simulink model "Problem3"  (R2020b)
settings: Solver=VariableStepAuto  StartTime=0.0  StopTime=120.0  RelTol=1e-3
settings Model: DataDictionary=Problem3.sldd  Creator=Shirish  LastModifiedBy=Shirish

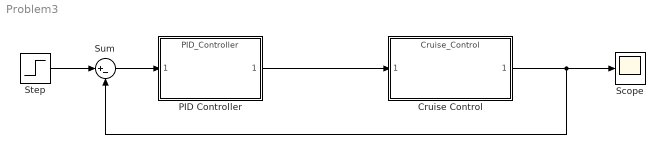
== system Problem3 ==
  Cruise Control : ModelReference  ModelNameDialog=Cruise_Control  SimulationMode=Normal  ModelReferenceVersion=1.15
  PID Controller : ModelReference  ModelNameDialog=PID_Controller  SimulationMode=Normal  ModelReferenceVersion=1.10
  Scope : Scope
  Step : Step  Time=0  SampleTime=0
  Sum : Sum  Inputs=|+-
  wires:
  Cruise Control/1 -> Sum/2, Scope/1
  Step/1 -> Sum/1
  PID Controller/1 -> Cruise Control/1
  Sum/1 -> PID Controller/1
